simulink model "control_structure_sim"  (R2014b)
settings: Solver=ode45  StartTime=0.0  StopTime=t_stop  RelTol=1e-3
undefined symbols (not defined in the file or in its folder): delta_a, delta_y, r_s, rho
libraries: cstblocks x2, simulink x1
settings Model: Creator=leliac  LastModifiedBy=leliac

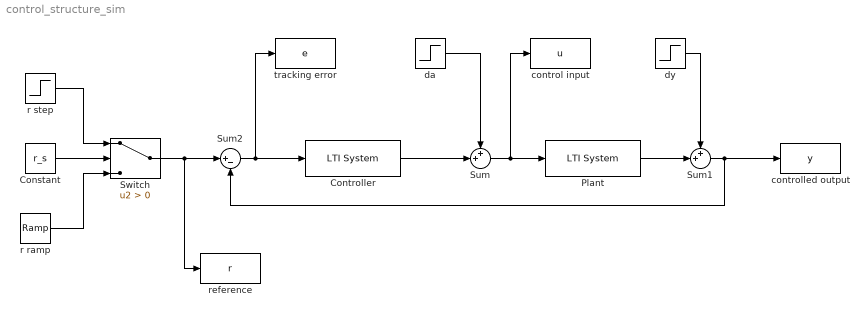
== system control_structure_sim ==
  Constant : Constant  Value=r_s
  Controller : cstblocks/LTI System  sys=C  IC=[]
  Plant : cstblocks/LTI System  sys=G  IC=[]
  Sum : Sum  Inputs=++|
  Sum1 : Sum  Inputs=++|
  Sum2 : Sum  Inputs=|+-
  Switch : Switch  Criteria=u2 > Threshold
  control input : ToWorkspace  VariableName=u  SaveFormat=Timeseries  SampleTime=-1
  "controlled output " : ToWorkspace  VariableName=y  SaveFormat=Timeseries  SampleTime=-1
  da : Step  Time=0  After=delta_a  SampleTime=0
  dy : Step  Time=0  After=delta_y  SampleTime=0
  r ramp : simulink/Sources/Ramp  slope=1  start=0  X0=0
  r step : Step  Time=0  After=rho  SampleTime=0
  reference : ToWorkspace  VariableName=r  SaveFormat=Timeseries  SampleTime=-1
  tracking error : ToWorkspace  VariableName=e  SaveFormat=Timeseries  SampleTime=-1
  wires:
  Controller/1 -> Sum/2
  Sum/1 -> control input/1, Plant/1
  Plant/1 -> Sum1/2
  Sum2/1 -> tracking error/1, Controller/1
  Sum1/1 -> Sum2/2, "controlled output "/1
  da/1 -> Sum/1
  dy/1 -> Sum1/1
  Switch/1 -> reference/1, Sum2/1
  Constant/1 -> Switch/2
  r step/1 -> Switch/1
  r ramp/1 -> Switch/3
